simulink model "vdPWalker_Belykh_etal_2016"  (R2022a)
settings: Solver=VariableStepAuto  StartTime=0.0  StopTime=10.0  RelTol=1e-3
settings Model: Creator=LEGION  LastModifiedBy=LEGION

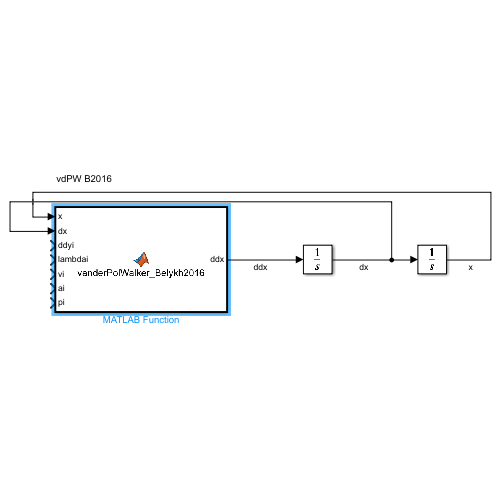
[thumbnail: Simulink's stored preview of the top-level diagram]
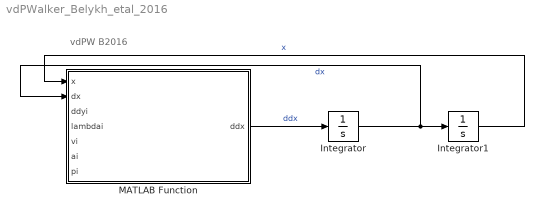
== system vdPWalker_Belykh_etal_2016 ==
  note: vdPW B2016
  Integrator : Integrator
  Integrator1 : Integrator
  MATLAB Function : MATLAB Function  TreatAsAtomicUnit=on
  wires:
  Integrator1/1 -> MATLAB Function/1(x)  "x"
  Integrator/1 -> Integrator1/1, MATLAB Function/2(dx)  "dx"
  MATLAB Function/1(ddx) -> Integrator/1  "ddx"

== matlab function vdPWalker_Belykh_etal_2016/MATLAB Function ==
  data: x input; ddx output; dx input; ddyi input; lambdai input; vi input; ai input; pi input
function ddx = vanderPolWalker_Belykh2016(x,dx,ddyi,lambdai,vi,ai,pi)
% Obtener aceleración del caminante según Belykh et al (2016)
% Alexis Contreras R. 

% Bistable gaits and wobbling induced by pedestrian-bridge interactions
% Igor V. Belykh, Russel Jeter and Vladimir N. Belykh (2016)

% Modelo de peatón de oscilador auto-sostenible donde los pasos se ajustan
% al movimiento del puente. El balance humano se modela como péndulo invertido.

%%%%%%%%%%%%%%%%%%%%%%%%%%%%%%%%%%%%%%%%%%%%%%%%%%%%%%%%%%%%%%%%%%%%%%%%%%%
% Inputs:
% x         -> Desplazamiento del centro de masa (CoM) del peatón
% dx        -> Velocidad del centro de masa del peatón 
% ddyi      -> Aceleración absoluta del puente (o relativa al suelo/punto fijo externo)
% lambdai   -> Parámetro de amortiguamiento
% vi        -> Parámetro de control del mecanismo de auto-excitación del caminar humano
% ai        -> Parámetro de control del mecanismo de auto-excitación del caminar humano
% pi        -> Desplazamiento horizontal del centro de presión del pie
% wi        -> wi = sqrt(g/L), del modelo pendulo invertido (L >> x)

% Outputs:
% ddx       -> Aceleración del peatón
%%%%%%%%%%%%%%%%%%%%%%%%%%%%%%%%%%%%%%%%%%%%%%%%%%%%%%%%%%%%%%%%%%%%%%%%%%%

sign_hat = sign(x);                                                         
if x == 0
    sign_hat = 1;                                                           
end

fxdx = lambdai*(dx^2+vi^2*(ai^2-(x-pi*sign_hat)^2))*dx - wi*(x-pi*sign_hat); % (Eq. 2)
ddx = -ddyi - fxdx;                                                         % (Eq. 1)
